simulink model "pacemaker_simulink"  (R2020a)
settings: Solver=FixedStepAuto  StartTime=0.0  StopTime=10.0  FixedStep=1e-3  RelTol=1e-3  EnableMultiTasking=on
undefined symbols (not defined in the file): A0, A1, D0, D1, D10, D11, D12, D13, D2, D3, D4, D5, D6, D7, D8, D9, PTA0, PTA1, PTA2, PTB2, PTB23, PTB3, PTB9, PTC16, PTC17, PTC2, PTC3, PTC4, PTD0, PTD1, PTD2, PTD3
libraries: frdmk64flib x19, etargetslib x2
settings Model: ExtModeTrigDuration=5  Creator=daniel  LastModifiedBy=daniel
settings OptimizationCC: EnhancedBackFolding=on  PassReuseOutputArgsAs=Individual arguments  ZeroExternalMemoryAtStartup=off  ZeroInternalMemoryAtStartup=off  MaxStackSize=64  OptimizeBlockOrder=speed  DifferentSizesBufferReuse=on  OptimizationCustomize=off  EfficientTunableParamExpr=on
settings DebuggingCC: ParameterTunabilityLossMsg=error
settings HardwareCC: ProdBitPerPointer=32  ProdBitPerSizeT=32  ProdBitPerPtrDiffT=32  ProdLargestAtomicInteger=Long  ProdLargestAtomicFloat=Double  ProdWordSize=32  ProdHWDeviceType=ARM Compatible->ARM Cortex
settings SFSimCC: MATLABDynamicMemAlloc=off
settings RTWCC: SystemTargetFile=ert.tlc  HardwareBoard=NXP FRDM-K64F  TemplateMakefile=ert_default_tmf  Toolchain=GNU Tools for ARM Embedded Processors
settings CodeAppCC: ForceParamTrailComments=on  IgnoreCustomStorageClasses=off  OperatorAnnotations=on  SimulinkDataObjDesc=on  SFDataObjDesc=on  InsertBlockDesc=on

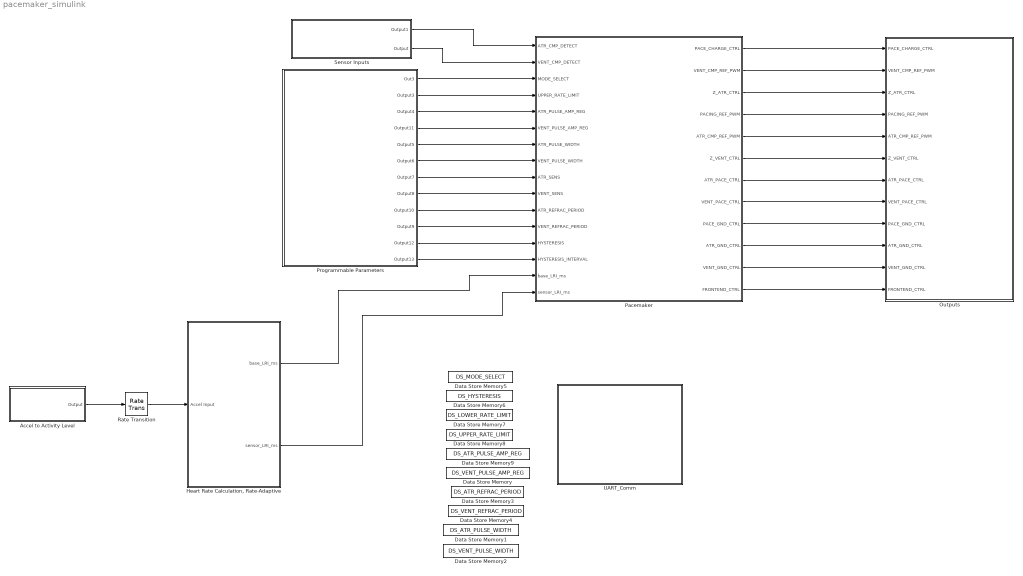
== system pacemaker_simulink ==
  Accel to Activity Level : Subsystem
  Data Store Memory : DataStoreMemory  DataStoreName=DS_VENT_PULSE_AMP_REG  ReadBeforeWriteMsg=warning  WriteAfterWriteMsg=warning  WriteAfterReadMsg=warning  InitialValue=3  ShowAdditionalParam=off
  Data Store Memory1 : DataStoreMemory  DataStoreName=DS_ATR_PULSE_WIDTH  ReadBeforeWriteMsg=warning  WriteAfterWriteMsg=warning  WriteAfterReadMsg=warning  InitialValue=40  ShowAdditionalParam=off
  Data Store Memory2 : DataStoreMemory  DataStoreName=DS_VENT_PULSE_WIDTH  ReadBeforeWriteMsg=warning  WriteAfterWriteMsg=warning  WriteAfterReadMsg=warning  InitialValue=40  ShowAdditionalParam=off
  Data Store Memory3 : DataStoreMemory  DataStoreName=DS_ATR_REFRAC_PERIOD  ReadBeforeWriteMsg=warning  WriteAfterWriteMsg=warning  WriteAfterReadMsg=warning  InitialValue=250  ShowAdditionalParam=off
  Data Store Memory4 : DataStoreMemory  DataStoreName=DS_VENT_REFRAC_PERIOD  ReadBeforeWriteMsg=warning  WriteAfterWriteMsg=warning  WriteAfterReadMsg=warning  InitialValue=320  ShowAdditionalParam=off
  Data Store Memory5 : DataStoreMemory  DataStoreName=DS_MODE_SELECT  ReadBeforeWriteMsg=warning  WriteAfterWriteMsg=warning  WriteAfterReadMsg=warning  ShowAdditionalParam=off
  Data Store Memory6 : DataStoreMemory  DataStoreName=DS_HYSTERESIS  ReadBeforeWriteMsg=warning  WriteAfterWriteMsg=warning  WriteAfterReadMsg=warning  InitialValue=false  ShowAdditionalParam=off
  Data Store Memory7 : DataStoreMemory  DataStoreName=DS_LOWER_RATE_LIMIT  ReadBeforeWriteMsg=warning  WriteAfterWriteMsg=warning  WriteAfterReadMsg=warning  InitialValue=60  ShowAdditionalParam=off
  Data Store Memory8 : DataStoreMemory  DataStoreName=DS_UPPER_RATE_LIMIT  ReadBeforeWriteMsg=warning  WriteAfterWriteMsg=warning  WriteAfterReadMsg=warning  InitialValue=150  ShowAdditionalParam=off
  Data Store Memory9 : DataStoreMemory  DataStoreName=DS_ATR_PULSE_AMP_REG  ReadBeforeWriteMsg=warning  WriteAfterWriteMsg=warning  WriteAfterReadMsg=warning  InitialValue=3  ShowAdditionalParam=off
  "Heart Rate Calculation, Rate-Adaptive" : Subsystem
  Outputs : Subsystem
  Pacemaker : Stateflow chart  TreatAsAtomicUnit=on
  Programmable Parameters : Subsystem
      settings: PortSchema="{\"entries\":[{\"content\":{\"sides\":[{\"content\":{\"connectorIds\":[]},\"type\":\"ConnectorPlacement.EquallySpacedRectSide\",\"uuid\":\"ad17499e-bbf1-46ac-9bc3-211a812e9102\"},{\"content\":{\"connectorIds\":[],\"side\":\"RIGHT\"},\"type\":\"ConnectorPlacement.EquallySpacedRectSide\",\"uuid\":\"568c1922-f5a0-4c26-aaad-185975cb380b\"},{\"content\":{\"connectorIds\":[],\"side\":\"TOP\"},\"type\":\"ConnectorPlacement.EquallySpacedRectSide\",\"uuid\":\"d207e90b-8621-47c5-8c13-82a36e9f435e\"},{\"content\":{\"connectorIds\":[\"Out1\",\"Out2\",\"Out3\",\"Out4\",\"Out5\",\"Out6\",\"Out7\",\"Out8\",\"Out9\",\"Out10\",\"Out11\",\"Out12\"],\"side\":\"BOTTOM\"},\"type\":\"ConnectorPlacement.EquallySpacedRectSide\",\"uuid\":\"3dce8df0-4d4b-4fe4-989f-5fe138a91413\"}]},\"type\":\"ConnectorPlacement.EquallySpacedConnector\",\"uuid\":\"338e4dbd-0331-4be2-9b95-53beecb91762\"}],\"packageUris\":[\"http://schema.mathworks.com/mf0/Connector/19700101\"],\"version\":\"1.0\"}"
  Rate Transition : RateTransition  OutPortSampleTime=0.001
  Sensor Inputs : Subsystem
  UART_Comm : Subsystem
  wires:
  Programmable Parameters/1(Out3) -> Pacemaker/3(MODE_SELECT)
  Programmable Parameters/2(Output3) -> Pacemaker/4(UPPER_RATE_LIMIT)
  Programmable Parameters/3(Output4) -> Pacemaker/5(ATR_PULSE_AMP_REG)
  Programmable Parameters/5(Output5) -> Pacemaker/7(ATR_PULSE_WIDTH)
  Programmable Parameters/4(Output11) -> Pacemaker/6(VENT_PULSE_AMP_REG)
  Programmable Parameters/6(Output6) -> Pacemaker/8(VENT_PULSE_WIDTH)
  Programmable Parameters/7(Output7) -> Pacemaker/9(ATR_SENS)
  Programmable Parameters/8(Output8) -> Pacemaker/10(VENT_SENS)
  Programmable Parameters/9(Output10) -> Pacemaker/11(ATR_REFRAC_PERIOD)
  Programmable Parameters/10(Output9) -> Pacemaker/12(VENT_REFRAC_PERIOD)
  Pacemaker/1(PACE_CHARGE_CTRL) -> Outputs/1(PACE_CHARGE_CTRL)
  Pacemaker/2(VENT_CMP_REF_PWM) -> Outputs/2(VENT_CMP_REF_PWM)
  Pacemaker/3(Z_ATR_CTRL) -> Outputs/3(Z_ATR_CTRL)
  Pacemaker/4(PACING_REF_PWM) -> Outputs/4(PACING_REF_PWM)
  Pacemaker/5(ATR_CMP_REF_PWM) -> Outputs/5(ATR_CMP_REF_PWM)
  Pacemaker/6(Z_VENT_CTRL) -> Outputs/6(Z_VENT_CTRL)
  Pacemaker/7(ATR_PACE_CTRL) -> Outputs/7(ATR_PACE_CTRL)
  Pacemaker/8(VENT_PACE_CTRL) -> Outputs/8(VENT_PACE_CTRL)
  Pacemaker/9(PACE_GND_CTRL) -> Outputs/9(PACE_GND_CTRL)
  Pacemaker/10(ATR_GND_CTRL) -> Outputs/10(ATR_GND_CTRL)
  Pacemaker/11(VENT_GND_CTRL) -> Outputs/11(VENT_GND_CTRL)
  Pacemaker/12(FRONTEND_CTRL) -> Outputs/12(FRONTEND_CTRL)
  Programmable Parameters/11(Output12) -> Pacemaker/13(HYSTERESIS)
  Programmable Parameters/12(Output13) -> Pacemaker/14(HYSTERESIS_INTERVAL)
  Sensor Inputs/1(Output1) -> Pacemaker/1(ATR_CMP_DETECT)
  Sensor Inputs/2(Output) -> Pacemaker/2(VENT_CMP_DETECT)
  "Heart Rate Calculation, Rate-Adaptive"/1(base_LRI_ms) -> Pacemaker/15(base_LRI_ms)
  "Heart Rate Calculation, Rate-Adaptive"/2(sensor_LRI_ms) -> Pacemaker/16(sensor_LRI_ms)
  Rate Transition/1 -> "Heart Rate Calculation, Rate-Adaptive"/1(Accel Input)
  Accel to Activity Level/1(Output) -> Rate Transition/1

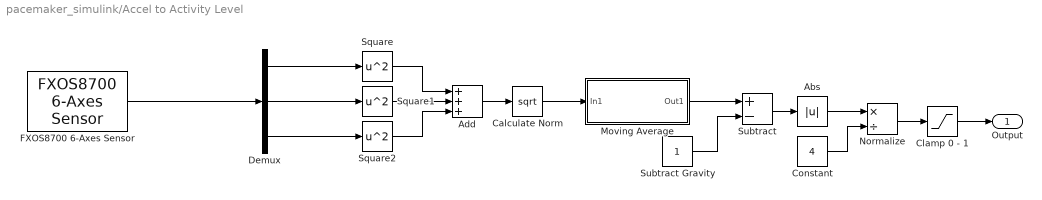
== system pacemaker_simulink/Accel to Activity Level ==
  Abs : Abs
  Add : Sum  Inputs=+++
  Calculate Norm : Sqrt  SaturateOnIntegerOverflow=on
  Clamp 0 - 1 : Saturate  UpperLimit=1  LowerLimit=0
  Constant : Constant  Value=4
  Demux : Demux  Outputs=3
  FXOS8700 6-Axes Sensor : frdmk64flib/FXOS8700 6-Axes Sensor  Activesensor=Accelerometer only  ODR=800Hz  HybridODR=400Hz  Accelfullrange=-4g to +4g  SampleTime=0.02
  Moving Average : Subsystem
  Normalize : Product  Inputs=*/
  Square : Math  Operator=square  SaturateOnIntegerOverflow=on
  Square1 : Math  Operator=square  SaturateOnIntegerOverflow=on
  Square2 : Math  Operator=square  SaturateOnIntegerOverflow=on
  Subtract : Sum  Inputs=+-
  Subtract Gravity : Constant
  Output : Outport
  wires:
  Subtract/1 -> Abs/1
  Square/1 -> Add/1
  Moving Average/1(Out1) -> Subtract/1
  Demux/1 -> Square/1
  Square1/1 -> Add/2
  Square2/1 -> Add/3
  Normalize/1 -> Clamp 0 - 1/1
  Abs/1 -> Normalize/1
  Add/1 -> Calculate Norm/1
  Calculate Norm/1 -> Moving Average/1(In1)
  Demux/2 -> Square1/1
  Demux/3 -> Square2/1
  Constant/1 -> Normalize/2
  Subtract Gravity/1 -> Subtract/2
  Clamp 0 - 1/1 -> Output/1
  FXOS8700 6-Axes Sensor/1 -> Demux/1

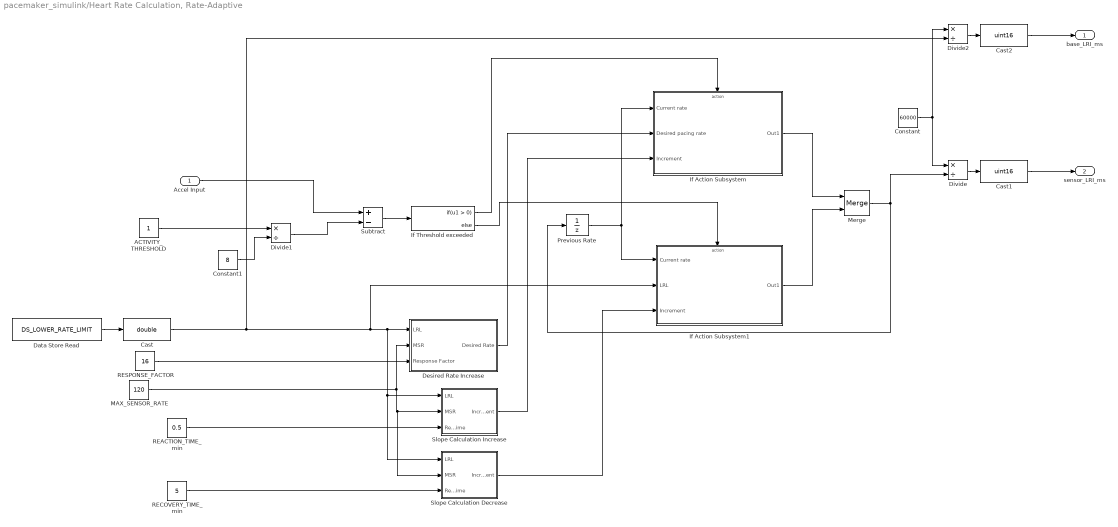
== system pacemaker_simulink/Heart Rate Calculation, Rate-Adaptive ==
  Accel Input : Inport
  ACTIVITY_THRESHOLD : Constant  OutDataTypeStr=double
  Cast : DataTypeConversion  OutDataTypeStr=double
  Cast1 : DataTypeConversion  OutDataTypeStr=uint16
  Cast2 : DataTypeConversion  OutDataTypeStr=uint16
  Constant : Constant  Value=60000
  Constant1 : Constant  Value=8
  Data Store Read : DataStoreRead  DataStoreName=DS_LOWER_RATE_LIMIT
  Desired Rate Increase : Subsystem
  Divide : Product  Inputs=*/
  Divide1 : Product  Inputs=*/
  Divide2 : Product  Inputs=*/
  If Action Subsystem : Subsystem  TreatAsAtomicUnit=on
  If Action Subsystem1 : Subsystem  TreatAsAtomicUnit=on
  If Threshold exceeded : If
  MAX_SENSOR_RATE : Constant  Value=120  OutDataTypeStr=double
  Merge : Merge
  Previous Rate : UnitDelay  InitialCondition=60  SampleTime=-1  HasFrameUpgradeWarning=on
  REACTION_TIME_min : Constant  Value=0.5
  RECOVERY_TIME_min : Constant  Value=5
  RESPONSE_FACTOR : Constant  Value=16  OutDataTypeStr=double
  Slope Calculation Decrease : Subsystem
  Slope Calculation Increase : Subsystem
  Subtract : Sum  Inputs=+-
  base_LRI_ms : Outport
  sensor_LRI_ms : Outport  Port=2
  wires:
  Desired Rate Increase/1(Desired Rate) -> If Action Subsystem/2(Desired pacing rate)
  Subtract/1 -> If Threshold exceeded/1
  Cast/1 -> Divide2/2, If Action Subsystem1/2(LRL), Slope Calculation Decrease/1(LRL), Slope Calculation Increase/1(LRL), Desired Rate Increase/1(LRL)
  MAX_SENSOR_RATE/1 -> Slope Calculation Decrease/2(MSR), Slope Calculation Increase/2(MSR), Desired Rate Increase/2(MSR)
  Previous Rate/1 -> If Action Subsystem1/1(Current rate), If Action Subsystem/1(Current rate)
  Accel Input/1 -> Subtract/1
  Merge/1 -> Divide/2, Previous Rate/1
  RESPONSE_FACTOR/1 -> Desired Rate Increase/3(Response Factor)
  REACTION_TIME_min/1 -> Slope Calculation Increase/3(ReactionTime)
  RECOVERY_TIME_min/1 -> Slope Calculation Decrease/3(RecoveryTime)
  Divide1/1 -> Subtract/2
  Constant1/1 -> Divide1/2
  ACTIVITY_THRESHOLD/1 -> Divide1/1
  Slope Calculation Decrease/1(Increment) -> If Action Subsystem1/3(Increment)
  Slope Calculation Increase/1(Increment) -> If Action Subsystem/3(Increment)
  If Threshold exceeded/1 -> If Action Subsystem/Action
  If Threshold exceeded/2 -> If Action Subsystem1/Action
  If Action Subsystem1/1(Out1) -> Merge/2
  If Action Subsystem/1(Out1) -> Merge/1
  Data Store Read/1 -> Cast/1
  Constant/1 -> Divide2/1, Divide/1
  Divide2/1 -> Cast2/1
  Divide/1 -> Cast1/1
  Cast1/1 -> sensor_LRI_ms/1
  Cast2/1 -> base_LRI_ms/1

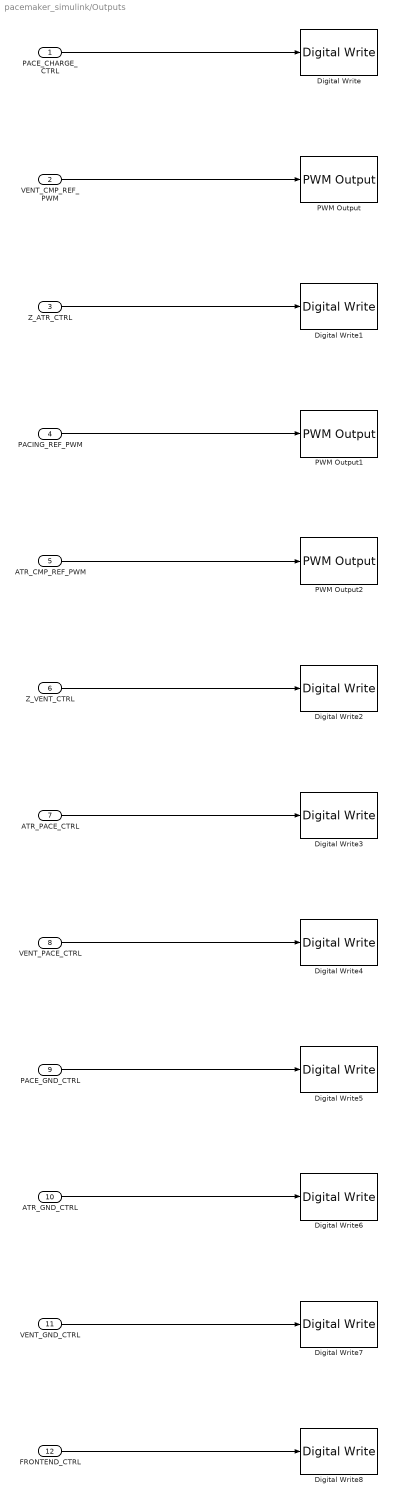
== system pacemaker_simulink/Outputs ==
  PACE_CHARGE_CTRL : Inport
  VENT_CMP_REF_PWM : Inport  Port=2
  Z_ATR_CTRL : Inport  Port=3
  PACING_REF_PWM : Inport  Port=4
  ATR_CMP_REF_PWM : Inport  Port=5
  Z_VENT_CTRL : Inport  Port=6
  ATR_PACE_CTRL : Inport  Port=7
  VENT_PACE_CTRL : Inport  Port=8
  PACE_GND_CTRL : Inport  Port=9
  ATR_GND_CTRL : Inport  Port=10
  VENT_GND_CTRL : Inport  Port=11
  FRONTEND_CTRL : Inport  Port=12
  Digital Write : frdmk64flib/Digital Write  Whichpin=PTB9 (D2)
  Digital Write1 : frdmk64flib/Digital Write  Whichpin=PTB23 (D4)
  Digital Write2 : frdmk64flib/Digital Write  Whichpin=PTC3 (D7)
  Digital Write3 : frdmk64flib/Digital Write  Whichpin=PTA0 (D8)
  Digital Write4 : frdmk64flib/Digital Write  Whichpin=PTC4 (D9)
  Digital Write5 : frdmk64flib/Digital Write  Whichpin=PTD0 (D10)
  Digital Write6 : frdmk64flib/Digital Write  Whichpin=PTD2 (D11)
  Digital Write7 : frdmk64flib/Digital Write  Whichpin=PTD3 (D12)
  Digital Write8 : frdmk64flib/Digital Write  Whichpin=PTD1 (D13)
  PWM Output : frdmk64flib/PWM Output  Whichpin=PTA1 (D3)  InitialFrequency=2000  InitialDutyCycle=0
  PWM Output1 : frdmk64flib/PWM Output  Whichpin=PTA2 (D5)  InitialFrequency=2000  InitialDutyCycle=0
  PWM Output2 : frdmk64flib/PWM Output  Whichpin=PTC2 (D6)  InitialFrequency=2000  InitialDutyCycle=0
  wires:
  PACE_CHARGE_CTRL/1 -> Digital Write/1
  VENT_CMP_REF_PWM/1 -> PWM Output/1
  Z_ATR_CTRL/1 -> Digital Write1/1
  PACING_REF_PWM/1 -> PWM Output1/1
  ATR_CMP_REF_PWM/1 -> PWM Output2/1
  Z_VENT_CTRL/1 -> Digital Write2/1
  ATR_PACE_CTRL/1 -> Digital Write3/1
  VENT_PACE_CTRL/1 -> Digital Write4/1
  PACE_GND_CTRL/1 -> Digital Write5/1
  ATR_GND_CTRL/1 -> Digital Write6/1
  VENT_GND_CTRL/1 -> Digital Write7/1
  FRONTEND_CTRL/1 -> Digital Write8/1

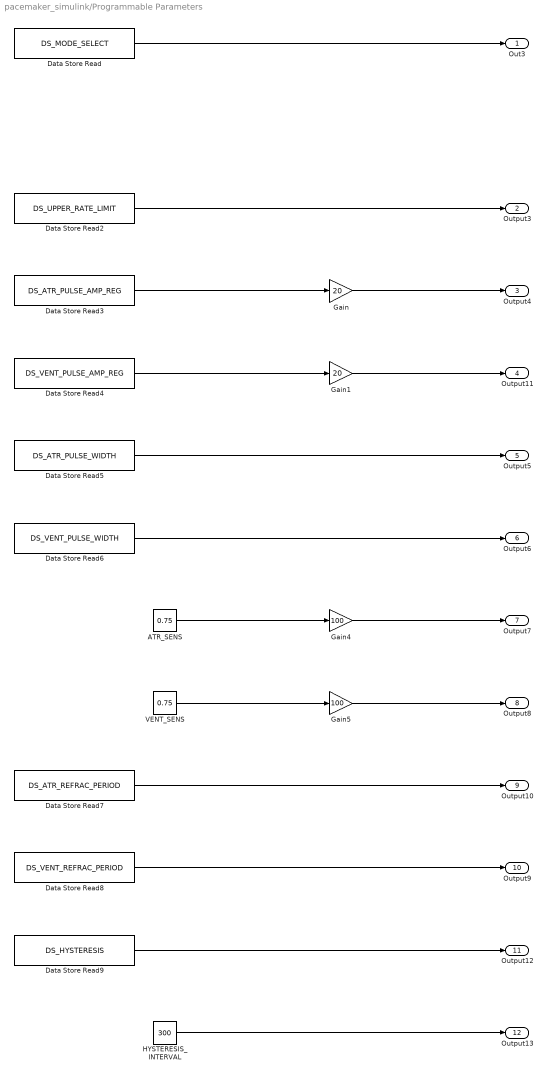
== system pacemaker_simulink/Programmable Parameters ==
  ATR_SENS : Constant  Value=0.75  OutDataTypeStr=double
  Data Store Read : DataStoreRead  DataStoreName=DS_MODE_SELECT
  Data Store Read2 : DataStoreRead  DataStoreName=DS_UPPER_RATE_LIMIT
  Data Store Read3 : DataStoreRead  DataStoreName=DS_ATR_PULSE_AMP_REG
  Data Store Read4 : DataStoreRead  DataStoreName=DS_VENT_PULSE_AMP_REG
  Data Store Read5 : DataStoreRead  DataStoreName=DS_ATR_PULSE_WIDTH
  Data Store Read6 : DataStoreRead  DataStoreName=DS_VENT_PULSE_WIDTH
  Data Store Read7 : DataStoreRead  DataStoreName=DS_ATR_REFRAC_PERIOD
  Data Store Read8 : DataStoreRead  DataStoreName=DS_VENT_REFRAC_PERIOD
  Data Store Read9 : DataStoreRead  DataStoreName=DS_HYSTERESIS
  Gain : Gain  Gain=20
  Gain1 : Gain  Gain=20
  Gain4 : Gain  Gain=100
  Gain5 : Gain  Gain=100
  HYSTERESIS_INTERVAL : Constant  Value=300  OutDataTypeStr=uint16
  VENT_SENS : Constant  Value=0.75  OutDataTypeStr=double
  Out3 : Outport
  Output3 : Outport  Port=2  Unit=ppm
  Output4 : Outport  Port=3  Unit=V
  Output11 : Outport  Port=4  Unit=V
  Output5 : Outport  Port=5  Unit=ms
  Output6 : Outport  Port=6  Unit=ms
  Output7 : Outport  Port=7  Unit=mV
  Output8 : Outport  Port=8  Unit=mV
  Output10 : Outport  Port=9  Unit=ms
  Output9 : Outport  Port=10  Unit=ms
  Output12 : Outport  Port=11
  Output13 : Outport  Port=12  Unit=ms
  wires:
  Data Store Read/1 -> Out3/1
  Gain/1 -> Output4/1
  ATR_SENS/1 -> Gain4/1
  Gain4/1 -> Output7/1
  Gain5/1 -> Output8/1
  VENT_SENS/1 -> Gain5/1
  Gain1/1 -> Output11/1
  HYSTERESIS_INTERVAL/1 -> Output13/1
  Data Store Read2/1 -> Output3/1
  Data Store Read3/1 -> Gain/1
  Data Store Read4/1 -> Gain1/1
  Data Store Read5/1 -> Output5/1
  Data Store Read6/1 -> Output6/1
  Data Store Read7/1 -> Output10/1
  Data Store Read8/1 -> Output9/1
  Data Store Read9/1 -> Output12/1

== system pacemaker_simulink/Sensor Inputs ==
  ATR_CMP_DETECT : frdmk64flib/Digital Read  Whichpin=PTC16 (D0)  SampleTime=-1
  VENT_CMP_DETECT : frdmk64flib/Digital Read  Whichpin=PTC17 (D1)  SampleTime=-1
  Output1 : Outport  OutDataTypeStr=boolean
  Output : Outport  Port=2  OutDataTypeStr=boolean
  wires:
  VENT_CMP_DETECT/1 -> Output/1
  ATR_CMP_DETECT/1 -> Output1/1

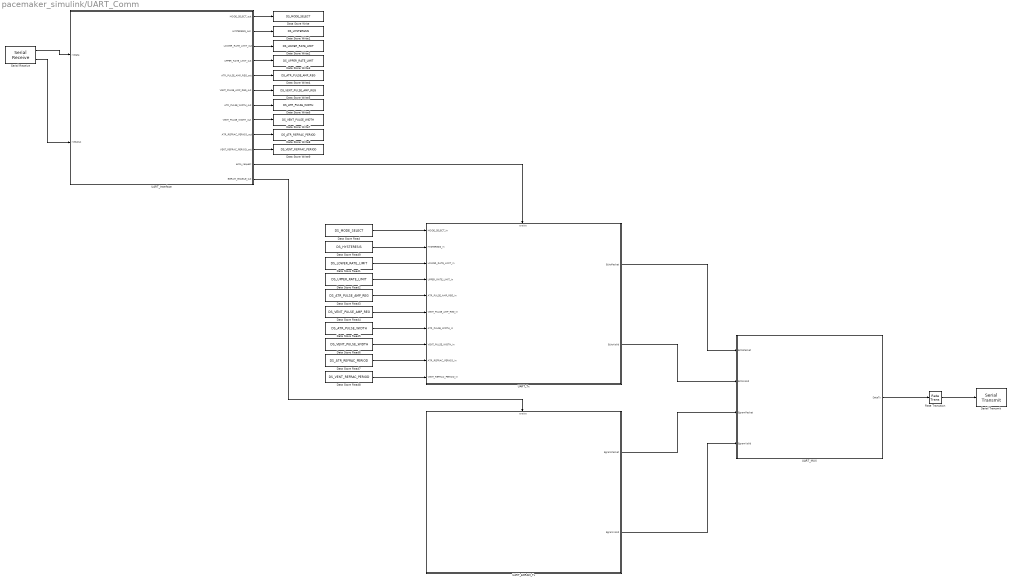
== system pacemaker_simulink/UART_Comm ==
  Data Store Read : DataStoreRead  DataStoreName=DS_MODE_SELECT
  Data Store Read1 : DataStoreRead  DataStoreName=DS_LOWER_RATE_LIMIT
  Data Store Read2 : DataStoreRead  DataStoreName=DS_UPPER_RATE_LIMIT
  Data Store Read3 : DataStoreRead  DataStoreName=DS_ATR_PULSE_AMP_REG
  Data Store Read4 : DataStoreRead  DataStoreName=DS_VENT_PULSE_AMP_REG
  Data Store Read5 : DataStoreRead  DataStoreName=DS_ATR_PULSE_WIDTH
  Data Store Read6 : DataStoreRead  DataStoreName=DS_VENT_PULSE_WIDTH
  Data Store Read7 : DataStoreRead  DataStoreName=DS_ATR_REFRAC_PERIOD
  Data Store Read8 : DataStoreRead  DataStoreName=DS_VENT_REFRAC_PERIOD
  Data Store Read9 : DataStoreRead  DataStoreName=DS_HYSTERESIS
  Data Store Write : DataStoreWrite  DataStoreName=DS_MODE_SELECT
  Data Store Write1 : DataStoreWrite  DataStoreName=DS_HYSTERESIS
  Data Store Write2 : DataStoreWrite  DataStoreName=DS_LOWER_RATE_LIMIT
  Data Store Write3 : DataStoreWrite  DataStoreName=DS_UPPER_RATE_LIMIT
  Data Store Write4 : DataStoreWrite  DataStoreName=DS_ATR_PULSE_AMP_REG
  Data Store Write5 : DataStoreWrite  DataStoreName=DS_VENT_PULSE_AMP_REG
  Data Store Write6 : DataStoreWrite  DataStoreName=DS_ATR_PULSE_WIDTH
  Data Store Write7 : DataStoreWrite  DataStoreName=DS_VENT_PULSE_WIDTH
  Data Store Write8 : DataStoreWrite  DataStoreName=DS_ATR_REFRAC_PERIOD
  Data Store Write9 : DataStoreWrite  DataStoreName=DS_VENT_REFRAC_PERIOD
  Rate Transition : RateTransition  OutPortSampleTime=0.005
  Serial Receive : frdmk64flib/Serial Receive  SCIModule=0  Baudrate=uint32(9600)  Parity=None  StopBits=1  HardwareFlowControl=None  ByteOrder=LittleEndian  DataType=uint8  DataLength=20  BlockingMode=off  OutputStatus=on  SampleTime=-1
  Serial Transmit : frdmk64flib/Serial Transmit  SCIModule=0  Baudrate=uint32(9600)  Parity=None  StopBits=1  HardwareFlowControl=None  ByteOrder=LittleEndian  BlockingMode=on  OutputStatus=off
  UART_EGRAM_Tx : Subsystem  TreatAsAtomicUnit=on
  UART_Interface : Stateflow chart  TreatAsAtomicUnit=on
  UART_MUX : Subsystem
  UART_Tx : Subsystem  TreatAsAtomicUnit=on
  wires:
  Serial Receive/1 -> UART_Interface/1(rxData)
  Serial Receive/2 -> UART_Interface/2(rxStatus)
  UART_Interface/2(HYSTERESIS_out) -> Data Store Write1/1
  UART_Interface/1(MODE_SELECT_out) -> Data Store Write/1
  UART_Interface/3(LOWER_RATE_LIMIT_out) -> Data Store Write2/1
  UART_Interface/4(UPPER_RATE_LIMIT_out) -> Data Store Write3/1
  UART_Interface/5(ATR_PULSE_AMP_REG_out) -> Data Store Write4/1
  UART_Interface/6(VENT_PULSE_AMP_REG_out) -> Data Store Write5/1
  UART_Interface/7(ATR_PULSE_WIDTH_out) -> Data Store Write6/1
  UART_Interface/8(VENT_PULSE_WIDTH_out) -> Data Store Write7/1
  UART_Interface/9(ATR_REFRAC_PERIOD_out) -> Data Store Write8/1
  UART_Interface/10(VENT_REFRAC_PERIOD_out) -> Data Store Write9/1
  Data Store Read/1 -> UART_Tx/1(MODE_SELECT_in)
  Data Store Read9/1 -> UART_Tx/2(HYSTERESIS_in)
  Data Store Read1/1 -> UART_Tx/3(LOWER_RATE_LIMIT_in)
  Data Store Read2/1 -> UART_Tx/4(UPPER_RATE_LIMIT_in)
  Data Store Read3/1 -> UART_Tx/5(ATR_PULSE_AMP_REG_in)
  Data Store Read4/1 -> UART_Tx/6(VENT_PULSE_AMP_REG_in)
  Data Store Read5/1 -> UART_Tx/7(ATR_PULSE_WIDTH_in)
  Data Store Read6/1 -> UART_Tx/8(VENT_PULSE_WIDTH_in)
  Data Store Read7/1 -> UART_Tx/9(ATR_REFRAC_PERIOD_in)
  Data Store Read8/1 -> UART_Tx/10(VENT_REFRAC_PERIOD_in)
  UART_Interface/11(echo_request) -> UART_Tx/Enable
  UART_Interface/12(EGRAM_ENABLE_out) -> UART_EGRAM_Tx/Enable
  UART_Tx/2(EchoValid) -> UART_MUX/2(EchoValid)
  UART_Tx/1(EchoPacket) -> UART_MUX/1(EchoPacket)
  UART_EGRAM_Tx/1(EgramPacket) -> UART_MUX/3(EgramPacket)
  UART_EGRAM_Tx/2(EgramValid) -> UART_MUX/4(EgramValid)
  Rate Transition/1 -> Serial Transmit/1
  UART_MUX/1(DataTx) -> Rate Transition/1

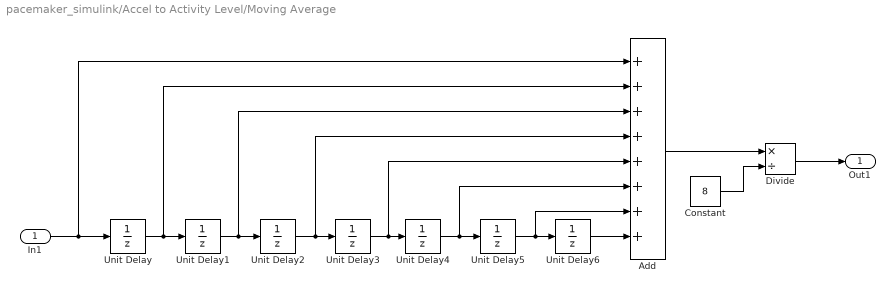
== system pacemaker_simulink/Accel to Activity Level/Moving Average ==
  In1 : Inport
  Add : Sum  Inputs=++++++++
  Constant : Constant  Value=8
  Divide : Product  Inputs=*/
  Unit Delay{,1..6} (7 alike) : UnitDelay  SampleTime=-1  HasFrameUpgradeWarning=on
  Out1 : Outport
  wires:
  In1/1 -> Add/1, Unit Delay/1
  Unit Delay/1 -> Add/2, Unit Delay1/1
  Unit Delay1/1 -> Add/3, Unit Delay2/1
  Unit Delay2/1 -> Add/4, Unit Delay3/1
  Unit Delay3/1 -> Add/5, Unit Delay4/1
  Unit Delay4/1 -> Add/6, Unit Delay5/1
  Unit Delay5/1 -> Add/7, Unit Delay6/1
  Unit Delay6/1 -> Add/8
  Add/1 -> Divide/1
  Divide/1 -> Out1/1
  Constant/1 -> Divide/2

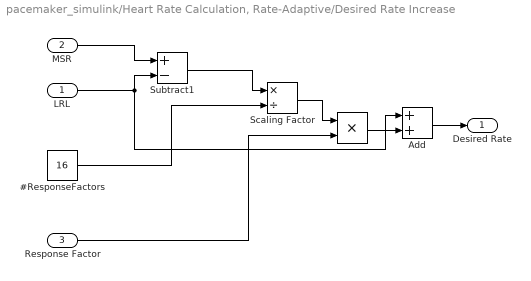
== system pacemaker_simulink/Heart Rate Calculation, Rate-Adaptive/Desired Rate Increase ==
  LRL : Inport
  MSR : Inport  Port=2
  Response Factor : Inport  Port=3
  " " : Product
  #ResponseFactors : Constant  Value=16
  Add : Sum
  Scaling Factor : Product  Inputs=*/
  Subtract1 : Sum  Inputs=+-
  Desired Rate : Outport
  wires:
  #ResponseFactors/1 -> Scaling Factor/2
  Subtract1/1 -> Scaling Factor/1
  MSR/1 -> Subtract1/1
  LRL/1 -> Add/1, Subtract1/2
  Scaling Factor/1 -> " "/1
  Response Factor/1 -> " "/2
  " "/1 -> Add/2
  Add/1 -> Desired Rate/1

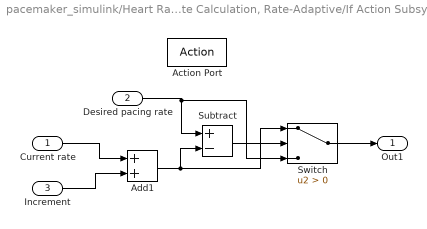
== system pacemaker_simulink/Heart Rate Calculation, Rate-Adaptive/If Action Subsystem ==
  Current rate : Inport
  Desired pacing rate : Inport  Port=2
  Increment : Inport  Port=3
  Action Port : ActionPort  ActionPortLabel=if(u1 > 0)
  Add1 : Sum
  Subtract : Sum  Inputs=+-
  Switch : Switch  Criteria=u2 > Threshold
  Out1 : Outport
  wires:
  Subtract/1 -> Switch/2
  Increment/1 -> Add1/2
  Switch/1 -> Out1/1
  Current rate/1 -> Add1/1
  Desired pacing rate/1 -> Switch/3, Subtract/1
  Add1/1 -> Switch/1, Subtract/2

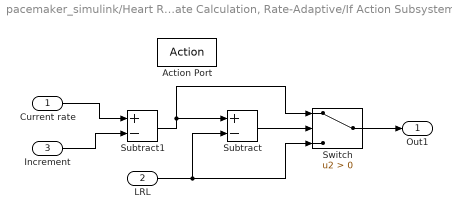
== system pacemaker_simulink/Heart Rate Calculation, Rate-Adaptive/If Action Subsystem1 ==
  Current rate : Inport
  LRL : Inport  Port=2
  Increment : Inport  Port=3
  Action Port : ActionPort  ActionPortLabel=else
  Subtract : Sum  Inputs=+-
  Subtract1 : Sum  Inputs=+-
  Switch : Switch  Criteria=u2 > Threshold
  Out1 : Outport
  wires:
  Switch/1 -> Out1/1
  LRL/1 -> Switch/3, Subtract/2
  Subtract/1 -> Switch/2
  Subtract1/1 -> Switch/1, Subtract/1
  Increment/1 -> Subtract1/2
  Current rate/1 -> Subtract1/1

== system pacemaker_simulink/Heart Rate Calculation, Rate-Adaptive/Slope Calculation Decrease ==
  LRL : Inport
  MSR : Inport  Port=2
  RecoveryTime : Inport  Port=3
  Constant : Constant  Value=1000
  Divide : Product  Inputs=*/
  Slope : Product  Inputs=*/
  Subtract1 : Sum  Inputs=+-
  Increment : Outport
  wires:
  Subtract1/1 -> Slope/1
  MSR/1 -> Subtract1/1
  RecoveryTime/1 -> Slope/2
  LRL/1 -> Subtract1/2
  Slope/1 -> Divide/1
  Constant/1 -> Divide/2
  Divide/1 -> Increment/1

== system pacemaker_simulink/Heart Rate Calculation, Rate-Adaptive/Slope Calculation Increase ==
  LRL : Inport
  MSR : Inport  Port=2
  ReactionTime : Inport  Port=3
  Constant : Constant  Value=1000
  Divide : Product  Inputs=*/
  Slope : Product  Inputs=*/
  Subtract1 : Sum  Inputs=+-
  Increment : Outport
  wires:
  Subtract1/1 -> Slope/1
  MSR/1 -> Subtract1/1
  ReactionTime/1 -> Slope/2
  LRL/1 -> Subtract1/2
  Slope/1 -> Divide/1
  Divide/1 -> Increment/1
  Constant/1 -> Divide/2

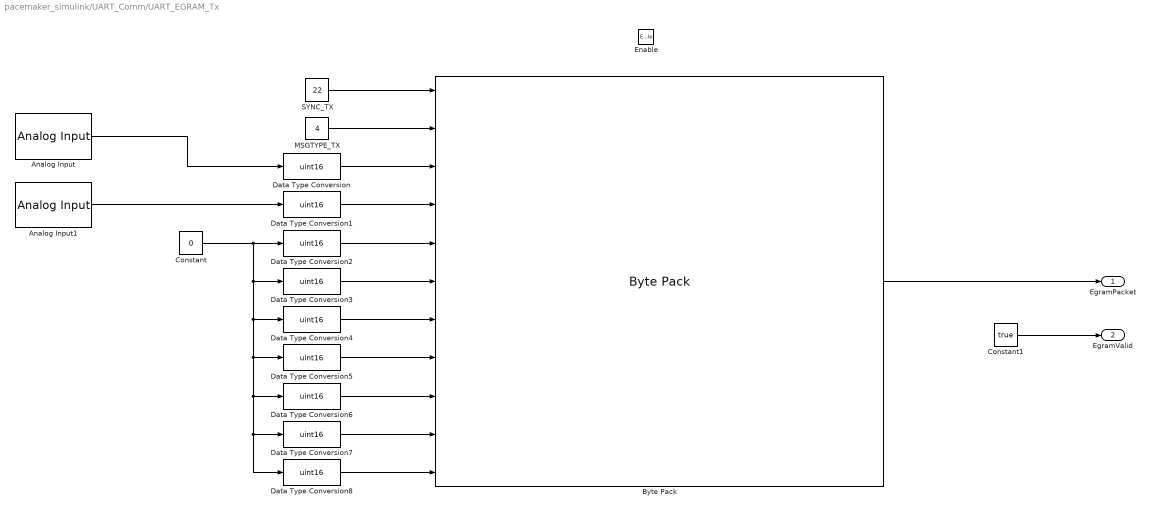
== system pacemaker_simulink/UART_Comm/UART_EGRAM_Tx ==
  Enable : EnablePort
  Analog Input : frdmk64flib/Analog Input  Whichpin=PTB2 (A0)  SampleTime=-1
  Analog Input1 : frdmk64flib/Analog Input  Whichpin=PTB3 (A1)  SampleTime=-1
  Byte Pack : etargetslib/Byte Pack  datatypes={'uint8','uint8','uint16','uint16', 'uint16','uint16','uint16','uint16', 'uint16','uint16','uint16'}  byteAlign=1
  Constant : Constant  Value=0
  Constant1 : Constant  Value=true
  Data Type Conversion{,1..8} (9 alike) : DataTypeConversion  OutDataTypeStr=uint16
  MSGTYPE_TX : Constant  Value=4  OutDataTypeStr=uint8
  SYNC_TX : Constant  Value=22  OutDataTypeStr=uint8
  EgramPacket : Outport  OutputWhenDisabled=reset  InitialOutput=0
  EgramValid : Outport  Port=2  OutputWhenDisabled=reset  InitialOutput=false
  wires:
  SYNC_TX/1 -> Byte Pack/1
  Data Type Conversion/1 -> Byte Pack/3
  Data Type Conversion2/1 -> Byte Pack/5
  Analog Input/1 -> Data Type Conversion/1
  Analog Input1/1 -> Data Type Conversion1/1
  MSGTYPE_TX/1 -> Byte Pack/2
  Data Type Conversion3/1 -> Byte Pack/6
  Data Type Conversion6/1 -> Byte Pack/9
  Data Type Conversion4/1 -> Byte Pack/7
  Data Type Conversion7/1 -> Byte Pack/10
  Data Type Conversion1/1 -> Byte Pack/4
  Data Type Conversion5/1 -> Byte Pack/8
  Byte Pack/1 -> EgramPacket/1
  Data Type Conversion8/1 -> Byte Pack/11
  Constant/1 -> Data Type Conversion8/1, Data Type Conversion7/1, Data Type Conversion6/1, Data Type Conversion5/1, Data Type Conversion4/1, Data Type Conversion3/1, Data Type Conversion2/1
  Constant1/1 -> EgramValid/1

== system pacemaker_simulink/UART_Comm/UART_MUX ==
  EchoPacket : Inport
  EchoValid : Inport  Port=2
  EgramPacket : Inport  Port=3
  EgramValid : Inport  Port=4
  Constant : Constant  Value=[0 0 0 0 0 0 0 0 0 0 0 0 0 0 0 0 0 0 0 0]  OutDataTypeStr=uint8
  Switch : Switch  Criteria=u2 > Threshold
  Switch1 : Switch  Criteria=u2 > Threshold
  DataTx : Outport
  wires:
  EgramPacket/1 -> Switch/1
  EchoPacket/1 -> Switch1/1
  EchoValid/1 -> Switch1/2
  EgramValid/1 -> Switch/2
  Constant/1 -> Switch/3
  Switch/1 -> Switch1/3
  Switch1/1 -> DataTx/1

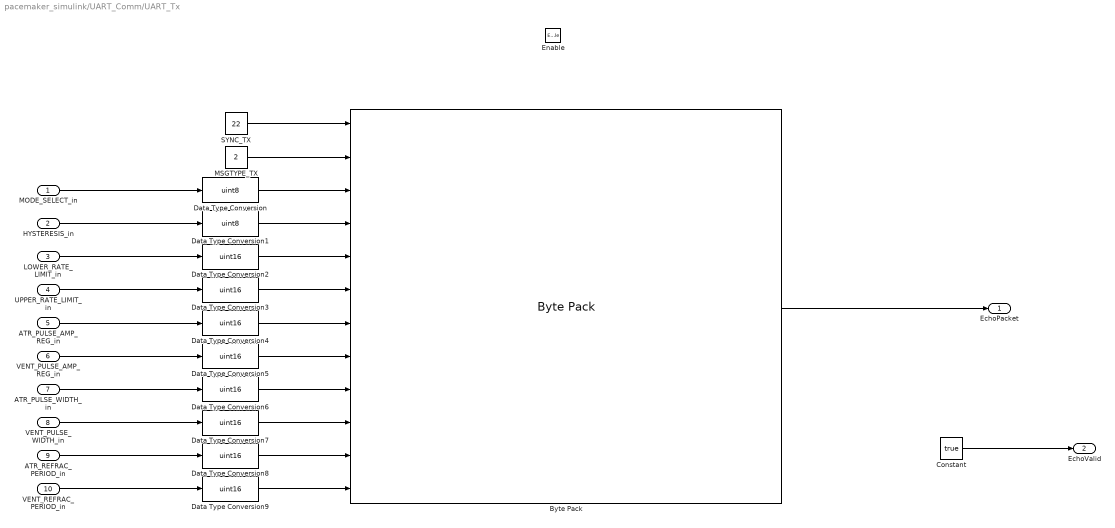
== system pacemaker_simulink/UART_Comm/UART_Tx ==
  MODE_SELECT_in : Inport
  HYSTERESIS_in : Inport  Port=2
  LOWER_RATE_LIMIT_in : Inport  Port=3
  UPPER_RATE_LIMIT_in : Inport  Port=4
  ATR_PULSE_AMP_REG_in : Inport  Port=5
  VENT_PULSE_AMP_REG_in : Inport  Port=6
  ATR_PULSE_WIDTH_in : Inport  Port=7
  VENT_PULSE_WIDTH_in : Inport  Port=8
  ATR_REFRAC_PERIOD_in : Inport  Port=9
  VENT_REFRAC_PERIOD_in : Inport  Port=10
  Enable : EnablePort
  Byte Pack : etargetslib/Byte Pack  datatypes={'uint8','uint8','uint8','uint8', 'uint16','uint16','uint16','uint16', 'uint16','uint16','uint16','uint16'}  byteAlign=1
  Constant : Constant  Value=true
  Data Type Conversion : DataTypeConversion  OutDataTypeStr=uint8
  Data Type Conversion1 : DataTypeConversion  OutDataTypeStr=uint8
  Data Type Conversion{2..9} (8 alike) : DataTypeConversion  OutDataTypeStr=uint16
  MSGTYPE_TX : Constant  Value=2  OutDataTypeStr=uint8
  SYNC_TX : Constant  Value=22  OutDataTypeStr=uint8
  EchoPacket : Outport  OutputWhenDisabled=reset  InitialOutput=0
  EchoValid : Outport  Port=2  OutputWhenDisabled=reset  InitialOutput=false
  wires:
  SYNC_TX/1 -> Byte Pack/1
  Data Type Conversion/1 -> Byte Pack/3
  Data Type Conversion2/1 -> Byte Pack/5
  VENT_REFRAC_PERIOD_in/1 -> Data Type Conversion9/1
  ATR_PULSE_WIDTH_in/1 -> Data Type Conversion6/1
  Data Type Conversion9/1 -> Byte Pack/12
  MODE_SELECT_in/1 -> Data Type Conversion/1
  HYSTERESIS_in/1 -> Data Type Conversion1/1
  LOWER_RATE_LIMIT_in/1 -> Data Type Conversion2/1
  VENT_PULSE_AMP_REG_in/1 -> Data Type Conversion5/1
  MSGTYPE_TX/1 -> Byte Pack/2
  Data Type Conversion3/1 -> Byte Pack/6
  Data Type Conversion6/1 -> Byte Pack/9
  Data Type Conversion4/1 -> Byte Pack/7
  UPPER_RATE_LIMIT_in/1 -> Data Type Conversion3/1
  ATR_REFRAC_PERIOD_in/1 -> Data Type Conversion8/1
  Data Type Conversion7/1 -> Byte Pack/10
  VENT_PULSE_WIDTH_in/1 -> Data Type Conversion7/1
  Data Type Conversion1/1 -> Byte Pack/4
  Data Type Conversion5/1 -> Byte Pack/8
  Byte Pack/1 -> EchoPacket/1
  Data Type Conversion8/1 -> Byte Pack/11
  ATR_PULSE_AMP_REG_in/1 -> Data Type Conversion4/1
  Constant/1 -> EchoValid/1

== stateflow chart pacemaker_simulink/UART_Comm/UART_Interface ==
  state SET
    entry:
    MODE_SELECT_out = rxData(3);
    HYSTERESIS_out = (rxData(4) ~= 0);
    LOWER_RATE_LIMIT_out = bitor( uint16(rxData(5)),  bitshift(uint16(rxData(6)), 8));
    UPPER_RATE_LIMIT_out = bitor( uint16(rxData(7)),  bitshift(uint16(rxData(8)), 8));
    ATR_PULSE_AMP_REG_out= bitor( uint16(rxData(9)),  bitshift(uint16(rxData(10)),8));
    VENT_PULSE_AMP_REG_out=bitor(uint16(rxData(11)), bitshift(uint16(rxData(12)),8));
    ATR_PULSE_WIDTH_out  = bitor( uint16(rxData(13)), bitshift(uint16(rxData(14)),8));
    VENT_PULSE_WIDTH_out = bitor( uint16(rxData(15)), bitshift(uint16(rxData(16)),8));
    ATR_REFRAC_PERIOD_out= bitor( uint16(rxData(17)), bitshift(uint16(rxData(18)),8));
    VENT_REFRAC_PERIOD_out=bitor(uint16(rxData(19)), bitshift(uint16(rxData(20)),8));
  state EGRAM_REQ
    entry:
    EGRAM_ENABLE_out = true;
  state INIT
    entry:
    MODE_SELECT_out = 0;    % AOO default
    HYSTERESIS_out = false;
    LOWER_RATE_LIMIT_out = 60;
    UPPER_RATE_LIMIT_out = 120;
    ATR_PULSE_AMP_REG_out = 4;
    VENT_PULSE_AMP_REG_out = 4;
    ATR_PULSE_WIDTH_out = 40;
    VENT_PULSE_WIDTH_out = 40;
    ATR_REFRAC_PERIOD_out = 250;
    VENT_REFRAC_PERIOD_out = 320;
    echo_request = false;
    EGRAM_ENABLE_out = false;
  state STANDBY
    entry:
    echo_request = false;
  state EGRAM_STOP
    EGRAM_ENABLE_out = false;
  state ECHO
    entry:
    echo_request = true;
  EGRAM_REQ -> STANDBY
  SET -> STANDBY
  (junction 29) -> EGRAM_REQ [order 3] : [rxData(2) == hex2dec('3')]
  (default) -> INIT
  (junction 29) -> SET [order 2] : [rxData(2) == hex2dec('1')]
  (junction 28) -> STANDBY [order 2]
  INIT -> STANDBY
  STANDBY -> (junction 28) : [rxStatus == 0]
  (junction 28) -> (junction 29) [order 1] : [rxData(1) == hex2dec('16')]
  (junction 29) -> EGRAM_STOP [order 4] : [rxData(2) == hex2dec('5')]
  (junction 29) -> ECHO [order 1] : [rxData(2) == hex2dec('2')]
  EGRAM_STOP -> STANDBY
  ECHO -> STANDBY : [after(500,msec)]
  data: rxData input uint8 size=20; rxStatus input uint8; MODE_SELECT_out output uint8; HYSTERESIS_out output boolean; LOWER_RATE_LIMIT_out output uint16; UPPER_RATE_LIMIT_out output uint16; ATR_PULSE_AMP_REG_out output uint16; VENT_PULSE_AMP_REG_out output uint16; ATR_PULSE_WIDTH_out output uint16; VENT_PULSE_WIDTH_out output uint16; ATR_REFRAC_PERIOD_out output uint16; VENT_REFRAC_PERIOD_out output uint16; echo_request output boolean; EGRAM_ENABLE_out output boolean

== stateflow chart pacemaker_simulink/Pacemaker ==
  state AOO
    during:
    if MODE_SELECT == 0 || MODE_SELECT == 1 || MODE_SELECT == 2 || MODE_SELECT == 3
    % Non-rate-adaptive modes: fixed LRL
    current_LRI_ms = base_LRI_ms;
    else
    % Rate-adaptive modes: use sensor-based rate
    current_LRI_ms = sensor_LRI_ms;
    end
    state Charging_and_Sensing
      entry:
      % Charging C22
      ATR_PACE_CTRL = 0;
      VENT_PACE_CTRL = 0;
      PACING_REF_PWM = ATR_PULSE_AMP_REG;
      PACE_CHARGE_CTRL = 1;
      % Discharging
      PACE_GND_CTRL = 1;
      VENT_PACE_CTRL = 0;
      Z_ATR_CTRL = 0;
      Z_VENT_CTRL = 0;
      ATR_PACE_CTRL = 0;
      ATR_GND_CTRL = 1;
      VENT_GND_CTRL = 0;
    state Pacing
      entry:
      % Pacing
      PACE_CHARGE_CTRL = 0;
      PACE_GND_CTRL = 1;
      ATR_PACE_CTRL = 1;
      ATR_GND_CTRL = 0;
      Z_ATR_CTRL = 0;
      Z_VENT_CTRL = 0;
      VENT_GND_CTRL = 0;
      VENT_PACE_CTRL = 0;
    note: Go into pacing after lower rate limit and upper rate limit has been reached
    note: Go back to charging/sensing after the pulse
    (default) -> AOO.Charging_and_Sensing
    AOO.Charging_and_Sensing -> AOO.Pacing : [after(current_LRI_ms - ATR_PULSE_WIDTH, msec)]
    AOO.Pacing -> AOO.Charging_and_Sensing : [after(ATR_PULSE_WIDTH, msec)]
  state VVI
    during:
    if MODE_SELECT == 0 || MODE_SELECT == 1 || MODE_SELECT == 2 || MODE_SELECT == 3
    % Non-rate-adaptive modes: fixed LRL
    current_LRI_ms = base_LRI_ms;
    else
    % Rate-adaptive modes: use sensor-based rate
    current_LRI_ms = sensor_LRI_ms;
    end
    note: If natural atrium beat detected, go back into charging and sensing state after refractory period
    state Pacing
      entry:
      FRONTEND_CTRL = 0;
      % Pacing
      PACE_CHARGE_CTRL = 0;
      PACE_GND_CTRL = 1;
      ATR_PACE_CTRL = 0;
      ATR_GND_CTRL = 0;
      Z_ATR_CTRL = 0;
      Z_VENT_CTRL = 0;
      VENT_GND_CTRL = 0;
      VENT_PACE_CTRL = 1;
    note: Go into pacing after lower rate limit has been reached
    state Charging_and_Sensing
      entry:
      FRONTEND_CTRL = 1;
      % Charging C22
      ATR_PACE_CTRL = 0;
      VENT_PACE_CTRL = 0;
      PACING_REF_PWM = VENT_PULSE_AMP_REG;
      PACE_CHARGE_CTRL = 1;
      % Discharging
      PACE_GND_CTRL = 1;
      VENT_PACE_CTRL = 0;
      Z_ATR_CTRL = 0;
      Z_VENT_CTRL = 0;
      ATR_PACE_CTRL = 0;
      ATR_GND_CTRL = 0;
      VENT_GND_CTRL = 1;
      VENT_CMP_REF_PWM = VENT_SENS;
    note: Go back to charging/sensing after the pulse
    state Hysteresis
      entry:
      FRONTEND_CTRL = 1;
      % Charging C22
      ATR_PACE_CTRL = 0;
      VENT_PACE_CTRL = 0;
      PACING_REF_PWM = VENT_PULSE_AMP_REG;
      PACE_CHARGE_CTRL = 1;
      % Discharging
      PACE_GND_CTRL = 1;
      VENT_PACE_CTRL = 0;
      Z_ATR_CTRL = 0;
      Z_VENT_CTRL = 0;
      ATR_PACE_CTRL = 0;
      ATR_GND_CTRL = 0;
      VENT_GND_CTRL = 1;
      VENT_CMP_REF_PWM = VENT_SENS;
    note: Go into pacing after lower rate limit with hysteresis delay has been reached
    note: If natural ventricular beat detected and hysteresis is active, go into hysteresis charging state
    note: If natural ventricular beat detected, go back into hysteresis charging and sensing state after refractory period
    (junction 117) -> (junction 120) : [after(VENT_PULSE_WIDTH, msec)]
    VVI.Charging_and_Sensing -> (junction 117) [order 3] : [HYSTERESIS == false && VENT_CMP_DETECT == 1]
    (junction 120) -> VVI.Charging_and_Sensing : [after(VENT_REFRAC_PERIOD, msec)]
    (default) -> VVI.Charging_and_Sensing
    VVI.Charging_and_Sensing -> VVI.Pacing [order 2] : [after(current_LRI_ms - VENT_PULSE_WIDTH, msec)]
    VVI.Pacing -> VVI.Charging_and_Sensing : [after(VENT_PULSE_WIDTH, msec)]
    VVI.Hysteresis -> VVI.Pacing [order 2] : [after(current_LRI_ms + HYSTERESIS_INTERVAL - VENT_PULSE_WIDTH, msec)]
    VVI.Charging_and_Sensing -> (junction 129) [order 1] : [HYSTERESIS == true && VENT_CMP_DETECT == 1]
    (junction 129) -> (junction 144) : [after(VENT_PULSE_WIDTH, msec)]
    (junction 144) -> VVI.Hysteresis : [after(VENT_REFRAC_PERIOD, msec)]
    VVI.Hysteresis -> (junction 134) [order 1] : [VENT_CMP_DETECT == 1]
    (junction 135) -> VVI.Hysteresis : [after(VENT_REFRAC_PERIOD, msec)]
    (junction 134) -> (junction 135) : [after(VENT_PULSE_WIDTH, msec)]
  state VOO
    during:
    if MODE_SELECT == 0 || MODE_SELECT == 1 || MODE_SELECT == 2 || MODE_SELECT == 3
    % Non-rate-adaptive modes: fixed LRL
    current_LRI_ms = base_LRI_ms;
    else
    % Rate-adaptive modes: use sensor-based rate
    current_LRI_ms = sensor_LRI_ms;
    end
    state Charging_and_Sensing
      entry:
      % Charging C22
      ATR_PACE_CTRL = 0;
      VENT_PACE_CTRL = 0;
      PACING_REF_PWM = VENT_PULSE_AMP_REG;
      PACE_CHARGE_CTRL = 1;
      % Discharging
      PACE_GND_CTRL = 1;
      VENT_PACE_CTRL = 0;
      Z_ATR_CTRL = 0;
      Z_VENT_CTRL = 0;
      ATR_PACE_CTRL = 0;
      ATR_GND_CTRL = 0;
      VENT_GND_CTRL = 1;
    note: Go into pacing after lower rate limit and upper rate limit has been reached
    state Pacing
      entry:
      % Pacing
      PACE_CHARGE_CTRL = 0;
      PACE_GND_CTRL = 1;
      ATR_PACE_CTRL = 0;
      ATR_GND_CTRL = 0;
      Z_ATR_CTRL = 0;
      Z_VENT_CTRL = 0;
      VENT_GND_CTRL = 0;
      VENT_PACE_CTRL = 1;
    note: Go back to charging/sensing after the pulse
    (default) -> VOO.Charging_and_Sensing
    VOO.Charging_and_Sensing -> VOO.Pacing : [after(current_LRI_ms - VENT_PULSE_WIDTH, msec)]
    VOO.Pacing -> VOO.Charging_and_Sensing : [after(VENT_PULSE_WIDTH, msec)]
  state Start
  state AAI
    during:
    if MODE_SELECT == 0 || MODE_SELECT == 1 || MODE_SELECT == 2 || MODE_SELECT == 3
    % Non-rate-adaptive modes: fixed LRL
    current_LRI_ms = base_LRI_ms;
    else
    % Rate-adaptive modes: use sensor-based rate
    current_LRI_ms = sensor_LRI_ms;
    end
    note: If natural atrium beat detected, go back into charging and sensing state after refractory period
    state Charging_and_Sensing
      entry:
      FRONTEND_CTRL = 1;
      % Charging C22
      ATR_PACE_CTRL = 0;
      VENT_PACE_CTRL = 0;
      PACING_REF_PWM = ATR_PULSE_AMP_REG;
      PACE_CHARGE_CTRL = 1;
      % Discharging
      PACE_GND_CTRL = 1;
      VENT_PACE_CTRL = 0;
      Z_ATR_CTRL = 0;
      Z_VENT_CTRL = 0;
      ATR_PACE_CTRL = 0;
      ATR_GND_CTRL = 1;
      VENT_GND_CTRL = 0;
      ATR_CMP_REF_PWM = ATR_SENS;
    state Pacing
      entry:
      FRONTEND_CTRL = 0;
      % Pacing
      PACE_CHARGE_CTRL = 0;
      PACE_GND_CTRL = 1;
      ATR_PACE_CTRL = 1;
      ATR_GND_CTRL = 0;
      Z_ATR_CTRL = 0;
      Z_VENT_CTRL = 0;
      VENT_GND_CTRL = 0;
      VENT_PACE_CTRL = 0;
    note: Go into pacing after lower rate limit has been reached
    note: Go back to charging/sensing after the pulse
    state Hysteresis
      entry:
      FRONTEND_CTRL = 1;
      % Charging C22
      ATR_PACE_CTRL = 0;
      VENT_PACE_CTRL = 0;
      PACING_REF_PWM = ATR_PULSE_AMP_REG;
      PACE_CHARGE_CTRL = 1;
      % Discharging
      PACE_GND_CTRL = 1;
      VENT_PACE_CTRL = 0;
      Z_ATR_CTRL = 0;
      Z_VENT_CTRL = 0;
      ATR_PACE_CTRL = 0;
      ATR_GND_CTRL = 1;
      VENT_GND_CTRL = 0;
      ATR_CMP_REF_PWM = ATR_SENS;
    note: Go into pacing after lower rate limit with hysteresis delay has been reached
    note: If natural atrium beat detected and hysteresis is active, go into hysteresis charging state
    note: If natural atrium beat detected, go back into hysteresis charging and sensing state after refractory period
    (junction 103) -> (junction 105) : [after(ATR_PULSE_WIDTH, msec)]
    AAI.Charging_and_Sensing -> (junction 103) [order 2] : [HYSTERESIS == false && ATR_CMP_DETECT == 1]
    (junction 105) -> AAI.Charging_and_Sensing : [after(ATR_REFRAC_PERIOD, msec)]
    (default) -> AAI.Charging_and_Sensing
    AAI.Charging_and_Sensing -> AAI.Pacing [order 1] : [after(current_LRI_ms - ATR_PULSE_WIDTH, msec)]
    AAI.Pacing -> AAI.Charging_and_Sensing : [after(ATR_PULSE_WIDTH, msec)]
    AAI.Charging_and_Sensing -> (junction 141) [order 3] : [HYSTERESIS == true && ATR_CMP_DETECT == 1]
    AAI.Hysteresis -> AAI.Pacing [order 2] : [after(current_LRI_ms + HYSTERESIS_INTERVAL - ATR_PULSE_WIDTH, msec)]
    (junction 141) -> (junction 146) : [after(ATR_PULSE_WIDTH, msec)]
    (junction 146) -> AAI.Hysteresis : [after(ATR_REFRAC_PERIOD, msec)]
    AAI.Hysteresis -> (junction 150) [order 1] : [ATR_CMP_DETECT == 1]
    (junction 151) -> AAI.Hysteresis : [after(ATR_REFRAC_PERIOD, msec)]
    (junction 150) -> (junction 151) : [after(ATR_PULSE_WIDTH, msec)]
  AOO -> Start : [MODE_SELECT ~= 0 && MODE_SELECT ~= 4]
  Start -> AOO [order 1] : [MODE_SELECT == 0 || MODE_SELECT == 4]
  (default) -> Start
  Start -> VVI [order 4] : [MODE_SELECT == 3 || MODE_SELECT == 7]
  Start -> VOO [order 2] : [MODE_SELECT == 1 || MODE_SELECT == 5]
  VVI -> Start : [MODE_SELECT ~= 3 && MODE_SELECT ~= 7]
  VOO -> Start : [MODE_SELECT ~= 1 && MODE_SELECT ~= 5]
  AAI -> Start : [MODE_SELECT ~= 2 && MODE_SELECT ~= 6]
  Start -> AAI [order 3] : [MODE_SELECT == 2 || MODE_SELECT == 6]
  data: ATR_CMP_DETECT input boolean; VENT_CMP_DETECT input boolean; MODE_SELECT input; UPPER_RATE_LIMIT input; ATR_PULSE_AMP_REG input; VENT_PULSE_AMP_REG input; ATR_PULSE_WIDTH input; VENT_PULSE_WIDTH input; ATR_SENS input; VENT_SENS input; ATR_REFRAC_PERIOD input; VENT_REFRAC_PERIOD input; PACE_CHARGE_CTRL output; VENT_CMP_REF_PWM output; Z_ATR_CTRL output; PACING_REF_PWM output; ATR_CMP_REF_PWM output; Z_VENT_CTRL output; ATR_PACE_CTRL output; VENT_PACE_CTRL output; PACE_GND_CTRL output; ATR_GND_CTRL output; VENT_GND_CTRL output; FRONTEND_CTRL output; HYSTERESIS input boolean; HYSTERESIS_INTERVAL input; base_LRI_ms input; sensor_LRI_ms input; current_LRI_ms local
